simulink model "Main"  (R2023a)
settings: Solver=ode4  StartTime=0.0  StopTime=inf  FixedStep=1e-5  RelTol=1e-3
libraries: canoelib x39, spsControlledVoltageSourceLib x3, spsCurrentMeasurementLib x3, slpidlib x2, vehdynlibsteering x1, spsPermanentMagnetSynchronousMachineLib x1, sps_lib x1, dspnetwork x1, etargetslib x1
settings Model: targetArch=x86  analysisModel=0  XcpMessageLength=-1  hasCAPLCallBlock=0  Creator=hatep  LastModifiedBy=hatep
settings RTWCC: Description=Vector CANoe Real-Time Target DLL (Visual C/C++ Project Makefile)  SystemTargetFile=cn.tlc  TemplateMakefile=cn_msdll.tmf
settings STFCustomTargetCC: ConcurrentExecutionCompliant=off  MatFileLogging=on  UseToolchainInfoCompliant=off  SystemTargetFile=cn.tlc
settings GRTTargetCC: ParMdlRefBuildCompliant=off  CompOptLevelCompliant=off  ConcurrentExecutionCompliant=off  CombineOutputUpdateFcns=off  CPPClassGenCompliant=off  GRTInterface=on  UseToolchainInfoCompliant=off  RTWCAPISignals=on  RTWCAPIParams=on

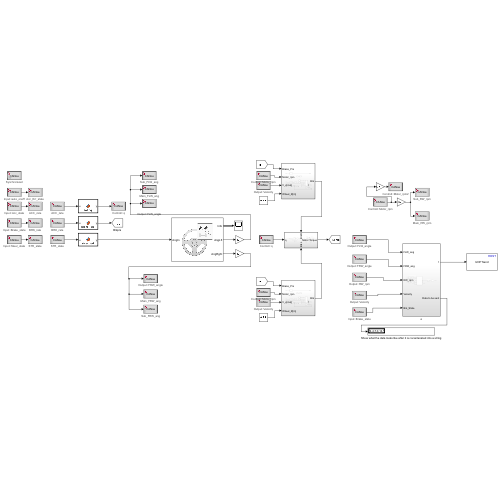
[thumbnail: Simulink's stored preview of the top-level diagram]
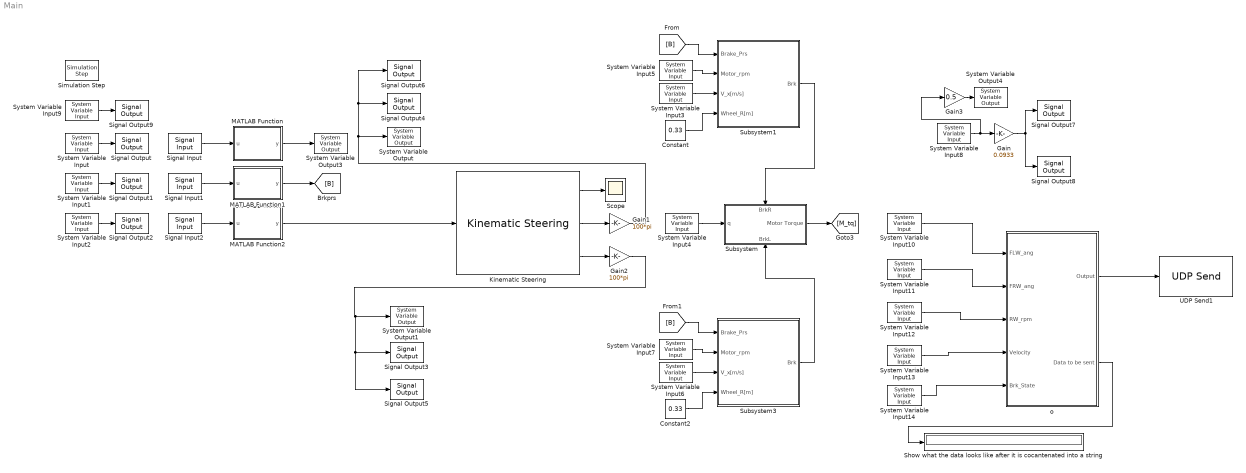
== system Main ==
  Constant : Constant  Value=0.33
  Constant2 : Constant  Value=0.33
  Gain : Gain  Gain=0.0933
  Gain1 : Gain  Gain=100*pi
  Gain2 : Gain  Gain=100*pi
  Gain3 : Gain  Gain=0.5
  Kinematic Steering : vehdynlibsteering/Kinematic Steering  StrgType=Ackerman  StrgRatioType=Constant  Loc=Front  NrmlFctr=1  TrckWdth=3  WhlBase=1.6  Db=0  StrgRng=3*pi  StrgAngBpts="[-6.2832   -5.0265   -3.7699   -2.5133   -1.2566         0    1.2566    2.5133    3.7699    5.0265    6.2832]"  StrgRatioTbl=|  StrgRatio=100  PctAckIn=off  PctAck=100  PctAckTbl=ones(1,11)*100  StrgArmLngth=0.1  RckCsLngth=0.5  TieRodLngth=0.248  D=0.2  PnnRadius=0.00085818  PnnRadiusTbl="[0.0055    0.0055    0.0056    0.0057    0.0058    0.0057    0.0057    0.0057    0.0056    0.0055    0.0055]"  RodLngth=0.1  ParaArmLngth=0.9  aMode=2
      | [13.5000   13.3750   13.2500   13.1250   13.0000   13.0000   13.0000   13.1250   13.2500   13.3750   13.5000
      | ]
  MATLAB Function : MATLAB Function  TreatAsAtomicUnit=on
  MATLAB Function1 : MATLAB Function  TreatAsAtomicUnit=on
  MATLAB Function2 : MATLAB Function  TreatAsAtomicUnit=on
  Scope : Scope
  Show what the data looks like after it is cocantenated into a string : Display
  Signal Input : canoelib/CANoe I//O/Signal Input  dbName=MBD  nodeName=Veh_Sim  msgName=Sim_1  sigName=ACC_rate  editSampleTime=0  rawValue=Default  dataType=Default  dataTypeDB=uint8  hasEncoding=off
      settings: AttributesFormatString=%<sigName>  SourceProductName=Vector CANoe
  Signal Input1 : canoelib/CANoe I//O/Signal Input  dbName=MBD  nodeName=Veh_Sim  msgName=Sim_1  sigName=BRK_rate  editSampleTime=0  rawValue=Default  dataType=Default  dataTypeDB=uint8  hasEncoding=off
      settings: AttributesFormatString=%<sigName>  SourceProductName=Vector CANoe
  Signal Input2 : canoelib/CANoe I//O/Signal Input  dbName=MBD  nodeName=Veh_Sim  msgName=Sim_1  sigName=STR_state  editSampleTime=0  rawValue=Default  dataType=Default  dataTypeDB=int8  hasEncoding=off
      settings: AttributesFormatString=%<sigName>  SourceProductName=Vector CANoe
  Signal Output : canoelib/CANoe I//O/Signal Output  dbName=MBD  nodeName=Veh_Sim  msgName=Sim_1  sigName=ACC_rate  rawValue=Default  dataType=Default  dataTypeDB=uint8  hasEncoding=off
      settings: AttributesFormatString=%<sigName>  SourceProductName=Vector CANoe
  Signal Output1 : canoelib/CANoe I//O/Signal Output  dbName=MBD  nodeName=Veh_Sim  msgName=Sim_1  sigName=BRK_rate  rawValue=Default  dataType=Default  dataTypeDB=uint8  hasEncoding=off
      settings: AttributesFormatString=%<sigName>  SourceProductName=Vector CANoe
  Signal Output2 : canoelib/CANoe I//O/Signal Output  dbName=MBD  nodeName=Veh_Sim  msgName=Sim_1  sigName=STR_state  rawValue=Default  dataType=Default  dataTypeDB=int8  hasEncoding=off
      settings: AttributesFormatString=%<sigName>  SourceProductName=Vector CANoe
  Signal Output3 : canoelib/CANoe I//O/Signal Output  dbName=MBD  nodeName=MainCtr  msgName=Ctr  sigName=Main_FRW_ang  rawValue=Raw value  dataType=Default  dataTypeDB=int8  hasEncoding=off
      settings: AttributesFormatString=%<sigName>  SourceProductName=Vector CANoe
  Signal Output4 : canoelib/CANoe I//O/Signal Output  dbName=MBD  nodeName=MainCtr  msgName=Ctr  sigName=Main_FLW_ang  rawValue=Raw value  dataType=Default  dataTypeDB=int8  hasEncoding=off
      settings: AttributesFormatString=%<sigName>  SourceProductName=Vector CANoe
  Signal Output5 : canoelib/CANoe I//O/Signal Output  dbName=MBD  nodeName=SubCtr  msgName=Sub_Ctr  sigName=Sub_FRW_ang  rawValue=Raw value  dataType=Default  dataTypeDB=uint8  hasEncoding=off
      settings: AttributesFormatString=%<sigName>  SourceProductName=Vector CANoe
  Signal Output6 : canoelib/CANoe I//O/Signal Output  dbName=MBD  nodeName=SubCtr  msgName=Sub_Ctr  sigName=Sub_FLW_ang  rawValue=Raw value  dataType=Default  dataTypeDB=uint8  hasEncoding=on
      settings: AttributesFormatString=%<sigName>  SourceProductName=Vector CANoe
  Signal Output7 : canoelib/CANoe I//O/Signal Output  dbName=MBD  nodeName=SubCtr  msgName=Sub_Ctr  sigName=Sub_RW_rpm  rawValue=Raw value  dataType=Default  dataTypeDB=uint16  hasEncoding=off
      settings: AttributesFormatString=%<sigName>  SourceProductName=Vector CANoe
  Signal Output8 : canoelib/CANoe I//O/Signal Output  dbName=MBD  nodeName=MainCtr  msgName=Ctr  sigName=Main_RW_rpm  rawValue=Raw value  dataType=Default  dataTypeDB=uint16  hasEncoding=off
      settings: AttributesFormatString=%<sigName>  SourceProductName=Vector CANoe
  Signal Output9 : canoelib/CANoe I//O/Signal Output  dbName=MBD  nodeName=Veh_Sim  msgName=Accel_Error_Condition  sigName=Acc_Err_state  rawValue=Default  dataType=Default  dataTypeDB=boolean  hasEncoding=off
      settings: AttributesFormatString=%<sigName>  SourceProductName=Vector CANoe
  Simulation Step : canoelib/CANoe I//O/Simulation Step  mode=Synchronized
      settings: AttributesFormatString=%<mode>  SourceProductName=Vector CANoe
  Subsystem : Subsystem
      settings: PortSchema="{\"entries\":[{\"content\":{\"sides\":[{\"content\":{\"connectorIds\":[\"In1\"]},\"type\":\"ConnectorPlacement.EquallySpacedRectSide\",\"uuid\":\"d856fc92-af2a-46c6-aa2d-f38a71ec206d\"},{\"content\":{\"connectorIds\":[\"Out1\"],\"side\":\"RIGHT\"},\"type\":\"ConnectorPlacement.EquallySpacedRectSide\",\"uuid\":\"749cbdd8-772b-4c60-b55a-bc78d69c198e\"},{\"content\":{\"connectorIds\":[\"In2\"],\"side\":\"TOP\"},\"type\":\"ConnectorPlacement.EquallySpacedRectSide\",\"uuid\":\"8a4e4948-29bd-4e64-b879-f0ed3d2cb3aa\"},{\"content\":{\"connectorIds\":[\"In3\"],\"side\":\"BOTTOM\"},\"type\":\"ConnectorPlacement.EquallySpacedRectSide\",\"uuid\":\"fb5f1ea8-5bd9-47f7-a40f-d5738de871d9\"}]},\"type\":\"ConnectorPlacement.EquallySpacedConnector\",\"uuid\":\"7c29b0f2-06f1-46e9-896a-7c6ebac9527c\"}],\"packageUris\":[\"http://schema.mathworks.com/mf0/Connector/R2020b\"],\"version\":\"1.0\"}"
  Subsystem1 : Subsystem
  Subsystem3 : Subsystem
  System Variable Input : canoelib/CANoe I//O/System Variable Input  nsName=Input  sysVarName=Acc_state  arrayIndex=-1  editSampleTime=0  rawValue=Default  dataType=Default  dataTypeDB=int32  hasEncoding=off  dataTypeCANoe=Get from CANoe
      settings: AttributesFormatString=%<nsName>::%<sysVarName>  SourceProductName=Vector CANoe
  System Variable Input1 : canoelib/CANoe I//O/System Variable Input  nsName=Input  sysVarName=Brake_state  arrayIndex=-1  editSampleTime=0  rawValue=Default  dataType=Default  dataTypeDB=int32  hasEncoding=off  dataTypeCANoe=Get from CANoe
      settings: AttributesFormatString=%<nsName>::%<sysVarName>  SourceProductName=Vector CANoe
  System Variable Input10 : canoelib/CANoe I//O/System Variable Input  nsName=Output  sysVarName=FLW_angle  arrayIndex=-1  editSampleTime=0  rawValue=Default  dataType=Default  dataTypeDB=int32  hasEncoding=off  dataTypeCANoe=Get from CANoe
      settings: AttributesFormatString=%<nsName>::%<sysVarName>  SourceProductName=Vector CANoe
  System Variable Input11 : canoelib/CANoe I//O/System Variable Input  nsName=Output  sysVarName=FRW_angle  arrayIndex=-1  editSampleTime=0  rawValue=Default  dataType=Default  dataTypeDB=int32  hasEncoding=off  dataTypeCANoe=Get from CANoe
      settings: AttributesFormatString=%<nsName>::%<sysVarName>  SourceProductName=Vector CANoe
  System Variable Input12 : canoelib/CANoe I//O/System Variable Input  nsName=Output  sysVarName=RW_rpm  arrayIndex=-1  editSampleTime=0  rawValue=Default  dataType=Default  dataTypeDB=int32  hasEncoding=off  dataTypeCANoe=Get from CANoe
      settings: AttributesFormatString=%<nsName>::%<sysVarName>  SourceProductName=Vector CANoe
  System Variable Input13 : canoelib/CANoe I//O/System Variable Input  nsName=Output  sysVarName=Velocity  arrayIndex=-1  editSampleTime=0  rawValue=Default  dataType=Default  dataTypeDB=int32  hasEncoding=off  dataTypeCANoe=Get from CANoe
      settings: AttributesFormatString=%<nsName>::%<sysVarName>  SourceProductName=Vector CANoe
  System Variable Input14 : canoelib/CANoe I//O/System Variable Input  nsName=Input  sysVarName=Brake_state  arrayIndex=-1  editSampleTime=0  rawValue=Default  dataType=Default  dataTypeDB=int32  hasEncoding=off  dataTypeCANoe=Get from CANoe
      settings: AttributesFormatString=%<nsName>::%<sysVarName>  SourceProductName=Vector CANoe
  System Variable Input2 : canoelib/CANoe I//O/System Variable Input  nsName=Input  sysVarName=Steer_state  arrayIndex=-1  editSampleTime=0  rawValue=Default  dataType=Default  dataTypeDB=int32  hasEncoding=off  dataTypeCANoe=Get from CANoe
      settings: AttributesFormatString=%<nsName>::%<sysVarName>  SourceProductName=Vector CANoe
  System Variable Input3 : canoelib/CANoe I//O/System Variable Input  nsName=Output  sysVarName=Velocity  arrayIndex=-1  editSampleTime=0  rawValue=Default  dataType=Default  dataTypeDB=int32  hasEncoding=off  dataTypeCANoe=Get from CANoe
      settings: AttributesFormatString=%<nsName>::%<sysVarName>  SourceProductName=Vector CANoe
  System Variable Input4 : canoelib/CANoe I//O/System Variable Input  nsName=Controll  sysVarName=q  arrayIndex=-1  editSampleTime=0  rawValue=Default  dataType=Default  dataTypeDB=double  hasEncoding=off  dataTypeCANoe=Get from CANoe
      settings: AttributesFormatString=%<nsName>::%<sysVarName>  SourceProductName=Vector CANoe
  System Variable Input5 : canoelib/CANoe I//O/System Variable Input  nsName=Controll  sysVarName=Motor_rpm  arrayIndex=-1  editSampleTime=0  rawValue=Default  dataType=Default  dataTypeDB=int32  hasEncoding=off  dataTypeCANoe=Get from CANoe
      settings: AttributesFormatString=%<nsName>::%<sysVarName>  SourceProductName=Vector CANoe
  System Variable Input6 : canoelib/CANoe I//O/System Variable Input  nsName=Output  sysVarName=Velocity  arrayIndex=-1  editSampleTime=0  rawValue=Default  dataType=Default  dataTypeDB=int32  hasEncoding=off  dataTypeCANoe=Get from CANoe
      settings: AttributesFormatString=%<nsName>::%<sysVarName>  SourceProductName=Vector CANoe
  System Variable Input7 : canoelib/CANoe I//O/System Variable Input  nsName=Controll  sysVarName=Motor_rpm  arrayIndex=-1  editSampleTime=0  rawValue=Default  dataType=Default  dataTypeDB=int32  hasEncoding=off  dataTypeCANoe=Get from CANoe
      settings: AttributesFormatString=%<nsName>::%<sysVarName>  SourceProductName=Vector CANoe
  System Variable Input8 : canoelib/CANoe I//O/System Variable Input  nsName=Controll  sysVarName=Motor_rpm  arrayIndex=-1  editSampleTime=0  rawValue=Default  dataType=Default  dataTypeDB=int32  hasEncoding=off  dataTypeCANoe=Get from CANoe
      settings: AttributesFormatString=%<nsName>::%<sysVarName>  SourceProductName=Vector CANoe
  System Variable Input9 : canoelib/CANoe I//O/System Variable Input  nsName=Input  sysVarName=auto_onoff  arrayIndex=-1  editSampleTime=0  rawValue=Default  dataType=Default  dataTypeDB=int32  hasEncoding=off  dataTypeCANoe=Get from CANoe
      settings: AttributesFormatString=%<nsName>::%<sysVarName>  SourceProductName=Vector CANoe
  System Variable Output : canoelib/CANoe I//O/System Variable Output  nsName=Output  sysVarName=FLW_angle  arrayIndex=-1  rawValue=Raw value  dataType=Default  dataTypeDB=int32  hasEncoding=off  dataTypeCANoe=Get from CANoe
      settings: AttributesFormatString=%<nsName>::%<sysVarName>  SourceProductName=Vector CANoe
  System Variable Output1 : canoelib/CANoe I//O/System Variable Output  nsName=Output  sysVarName=FRW_angle  arrayIndex=-1  rawValue=Raw value  dataType=Default  dataTypeDB=int32  hasEncoding=off  dataTypeCANoe=Get from CANoe
      settings: AttributesFormatString=%<nsName>::%<sysVarName>  SourceProductName=Vector CANoe
  System Variable Output3 : canoelib/CANoe I//O/System Variable Output  nsName=Controll  sysVarName=q  arrayIndex=-1  rawValue=Default  dataType=Default  dataTypeDB=double  hasEncoding=off  dataTypeCANoe=Get from CANoe
      settings: AttributesFormatString=%<nsName>::%<sysVarName>  SourceProductName=Vector CANoe
  System Variable Output4 : canoelib/CANoe I//O/System Variable Output  nsName=Controll  sysVarName=Motor_rpm2  arrayIndex=-1  rawValue=Raw value  dataType=Default  dataTypeDB=int32  hasEncoding=off  dataTypeCANoe=Get from CANoe
      settings: AttributesFormatString=%<nsName>::%<sysVarName>  SourceProductName=Vector CANoe
  UDP Send1 : dspnetwork/UDP Send  remoteURL='127.0.0.1'  remotePort=25000  localURL='0.0.0.0'  localPortSource=Automatically determine  localPort=-1  sendBufferSize=8192  sampletime=-1  blockPlatform=HOST  separateLengthPort=0
  o : Subsystem
  wires:
  MATLAB Function/1(y) -> System Variable Output3/1
  MATLAB Function1/1(y) -> [B]
  Kinematic Steering/2 -> Gain1/1
  Kinematic Steering/3 -> Gain2/1
  Kinematic Steering/1 -> Scope/1
  MATLAB Function2/1(y) -> Kinematic Steering/1
  System Variable Input/1 -> Signal Output/1
  Signal Input/1 -> MATLAB Function/1(u)
  Signal Input1/1 -> MATLAB Function1/1(u)
  Signal Input2/1 -> MATLAB Function2/1(u)
  System Variable Input1/1 -> Signal Output1/1
  System Variable Input2/1 -> Signal Output2/1
  Gain1/1 -> Signal Output6/1, Signal Output4/1, System Variable Output/1
  Gain2/1 -> Signal Output5/1, Signal Output3/1, System Variable Output1/1
  System Variable Input4/1 -> Subsystem/1(q)
  Subsystem/1(Motor Torque) -> [M_tq]
  Constant/1 -> Subsystem1/4(Wheel_R[m])
  [B] -> Subsystem1/1(Brake_Prs)
  System Variable Input3/1 -> Subsystem1/3(V_x[m/s])
  System Variable Input5/1 -> Subsystem1/2(Motor_rpm)
  Subsystem1/1(Brk) -> Subsystem/2(BrkR)
  System Variable Input7/1 -> Subsystem3/2(Motor_rpm)
  System Variable Input6/1 -> Subsystem3/3(V_x[m/s])
  [B] -> Subsystem3/1(Brake_Prs)
  Constant2/1 -> Subsystem3/4(Wheel_R[m])
  Subsystem3/1(Brk) -> Subsystem/3(BrkL)
  System Variable Input8/1 -> Gain3/1, Gain/1
  Gain/1 -> Signal Output7/1, Signal Output8/1
  Gain3/1 -> System Variable Output4/1
  o/1(Output) -> UDP Send1/1
  o/2(Data to be sent) -> Show what the data looks like after it is cocantenated into a string/1
  System Variable Input10/1 -> o/1(FLW_ang)
  System Variable Input11/1 -> o/2(FRW_ang)
  System Variable Input12/1 -> o/3(RW_rpm)
  System Variable Input13/1 -> o/4(Velocity)
  System Variable Input14/1 -> o/5(Brk_State)
  System Variable Input9/1 -> Signal Output9/1

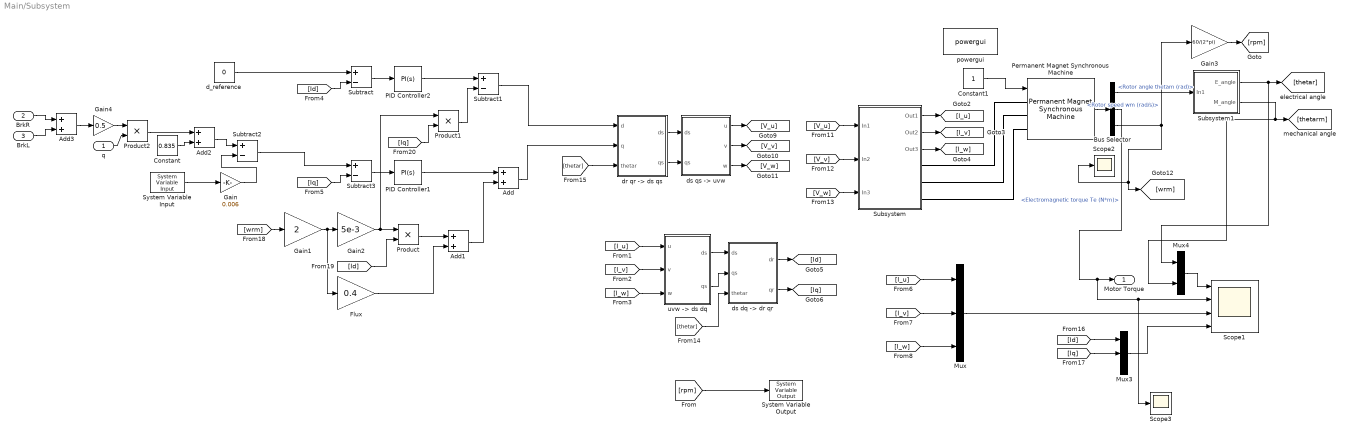
== system Main/Subsystem ==
  q : Inport
  BrkR : Inport  Port=2
  BrkL : Inport  Port=3
  Add{,1..3} (4 alike) : Sum
  Bus Selector : BusSelector  OutputSignals=Rotor angle thetam (rad),Electromagnetic torque Te (N*m),Rotor speed wm (rad/s)
  Constant : Constant  Value=0.835
  Constant1 : Constant
  Flux : Gain  Gain=0.4
  Gain : Gain  Gain=0.006
  Gain1 : Gain  Gain=2
  Gain2 : Gain  Gain=5e-3
  Gain3 : Gain  Gain=60/(2*pi)
  Gain4 : Gain  Gain=0.5
  Mux : Mux  Inputs=3
  Mux3 : Mux  Inputs=3
  Mux4 : Mux  Inputs=2
  PID Controller1 : slpidlib/PID Controller  Controller=PI  Form=Parallel  TimeDomain=Continuous-time  UseExternalTs=off  SampleTime=-1  IntegratorMethod=Forward Euler  FilterMethod=Forward Euler  ControllerParametersSource=internal  P=0.005*500*2*pi  I=0.5*500*2*pi  UseKiTs=off  D=0  N=100  UseFilter=on  TunerSelectOption=Transfer Function Based (PID Tuner App)  InitialConditionSource=internal  InitialConditionForIntegrator=0  InitialConditionForFilter=0  DifferentiatorICPrevScaledInput=0  ExternalReset=none  TrackingMode=off  Kt=1  LimitOutput=off  SatLimitsSource=internal  UpperSaturationLimit=inf  LowerSaturationLimit=-inf  LinearizeAsGain=on  AntiWindupMode=none  Kb=1  LimitIntegrator=off  UpperIntegratorSaturationLimit=inf  LowerIntegratorSaturationLimit=-inf  POutMin=[]  POutMax=[]  IOutMin=[]  IOutMax=[]  DOutMin=[]  DOutMax=[]  NOutMin=[]  NOutMax=[]  SumOutMin=[]  SumOutMax=[]  SaturationOutMin=[]  SaturationOutMax=[]  PParamMin=[]  PParamMax=[]  IParamMin=[]  IParamMax=[]  DParamMin=[]  DParamMax=[]  NParamMin=[]  NParamMax=[]  KbParamMin=[]  KbParamMax=[]  KtParamMin=[]  KtParamMax=[]  KbOutMin=[]  KbOutMax=[]  KtOutMin=[]  KtOutMax=[]  IntegratorOutMin=[]  IntegratorOutMax=[]  FilterOutMin=[]  FilterOutMax=[]  SumI1OutMin=[]  SumI1OutMax=[]  SumI2OutMin=[]  SumI2OutMax=[]  SumI3OutMin=[]  SumI3OutMax=[]  SumI4OutMin=[]  SumI4OutMax=[]  SumDOutMin=[]  SumDOutMax=[]  DifferentiatorOutMin=[]  DifferentiatorOutMax=[]  FilterDiffOutCoefMin=[]  FilterDiffOutCoefMax=[]  ReciprocalOutMin=[]  ReciprocalOutMax=[]  SumDenOutMin=[]  SumDenOutMax=[]  SumNumOutMin=[]  SumNumOutMax=[]  DivideOutMin=[]  DivideOutMax=[]  UdiffTsProdOutMin=[]  UdiffTsProdOutMax=[]  NTsProdOutMin=[]  NTsProdOutMax=[]  UintegralTsProdOutMin=[]  UintegralTsProdOutMax=[]  UngainTsProdOutMin=[]  UngainTsProdOutMax=[]  ClampingZeroOutDataTypeStr=Inherit: Inherit via back propagation  ClampingZeroOutMin=[]  ClampingZeroOutMax=[]  FilterDenConstantOutDataTypeStr=Inherit: Inherit via back propagation  FilterDenConstantOutMin=[]  FilterDenConstantOutMax=[]  PCopyOutDataTypeStr=Inherit: Inherit via back propagation  PCopyOutMin=[]  PCopyOutMax=[]  NCopyOutDataTypeStr=Inherit: Inherit via back propagation  NCopyOutMin=[]  NCopyOutMax=[]  IntegratorContinuousStateAttributes=''  IntegratorStateMustResolveToSignalObject=off  IntegratorRTWStateStorageClass=Auto  FilterContinuousStateAttributes=''  FilterStateMustResolveToSignalObject=off  FilterRTWStateStorageClass=Auto  ParallelPVariant=InternalParameters  IdealPVariant=Disabled  IVariant=InternalParameters  DVariant=Disabled  IntegratorVariant=Continuous  SatVariant=Disabled  AWVariant=Passthrough  PCopyVariant=Disabled  TRVariant=Disabled  FdbkBlocksVariant=Forward  IdealPFdbkVariant=Disabled  SatFdbkVariant=Disabled  DerivativeFilterVariant=Disabled  NVariant=Disabled  NCopyVariant=Disabled_SignalSpec  FilterICVariant=Disabled  IntegratorICVariant=InternalICs  ExternalResetVariant=Disabled  TRSumVariant=Passthrough  SumFdbkVariant=Disabled  SumVariant=Sum_PI  TsampFilterVariant=InternalTs  TsampNgainVariant=Passthrough  TsampIntegralVariant=Disabled_SignalSpec  ExternalSaturationOutDataTypeStr=Inherit: Same as second input
  PID Controller2 : slpidlib/PID Controller  Controller=PI  Form=Parallel  TimeDomain=Continuous-time  UseExternalTs=off  SampleTime=-1  IntegratorMethod=Forward Euler  FilterMethod=Forward Euler  ControllerParametersSource=internal  P=0.005*500*2*pi  I=0.5*500*2*pi  UseKiTs=off  D=0  N=100  UseFilter=on  TunerSelectOption=Transfer Function Based (PID Tuner App)  InitialConditionSource=internal  InitialConditionForIntegrator=0  InitialConditionForFilter=0  DifferentiatorICPrevScaledInput=0  ExternalReset=none  TrackingMode=off  Kt=1  LimitOutput=off  SatLimitsSource=internal  UpperSaturationLimit=inf  LowerSaturationLimit=-inf  LinearizeAsGain=on  AntiWindupMode=none  Kb=1  LimitIntegrator=off  UpperIntegratorSaturationLimit=inf  LowerIntegratorSaturationLimit=-inf  POutMin=[]  POutMax=[]  IOutMin=[]  IOutMax=[]  DOutMin=[]  DOutMax=[]  NOutMin=[]  NOutMax=[]  SumOutMin=[]  SumOutMax=[]  SaturationOutMin=[]  SaturationOutMax=[]  PParamMin=[]  PParamMax=[]  IParamMin=[]  IParamMax=[]  DParamMin=[]  DParamMax=[]  NParamMin=[]  NParamMax=[]  KbParamMin=[]  KbParamMax=[]  KtParamMin=[]  KtParamMax=[]  KbOutMin=[]  KbOutMax=[]  KtOutMin=[]  KtOutMax=[]  IntegratorOutMin=[]  IntegratorOutMax=[]  FilterOutMin=[]  FilterOutMax=[]  SumI1OutMin=[]  SumI1OutMax=[]  SumI2OutMin=[]  SumI2OutMax=[]  SumI3OutMin=[]  SumI3OutMax=[]  SumI4OutMin=[]  SumI4OutMax=[]  SumDOutMin=[]  SumDOutMax=[]  DifferentiatorOutMin=[]  DifferentiatorOutMax=[]  FilterDiffOutCoefMin=[]  FilterDiffOutCoefMax=[]  ReciprocalOutMin=[]  ReciprocalOutMax=[]  SumDenOutMin=[]  SumDenOutMax=[]  SumNumOutMin=[]  SumNumOutMax=[]  DivideOutMin=[]  DivideOutMax=[]  UdiffTsProdOutMin=[]  UdiffTsProdOutMax=[]  NTsProdOutMin=[]  NTsProdOutMax=[]  UintegralTsProdOutMin=[]  UintegralTsProdOutMax=[]  UngainTsProdOutMin=[]  UngainTsProdOutMax=[]  ClampingZeroOutDataTypeStr=Inherit: Inherit via back propagation  ClampingZeroOutMin=[]  ClampingZeroOutMax=[]  FilterDenConstantOutDataTypeStr=Inherit: Inherit via back propagation  FilterDenConstantOutMin=[]  FilterDenConstantOutMax=[]  PCopyOutDataTypeStr=Inherit: Inherit via back propagation  PCopyOutMin=[]  PCopyOutMax=[]  NCopyOutDataTypeStr=Inherit: Inherit via back propagation  NCopyOutMin=[]  NCopyOutMax=[]  IntegratorContinuousStateAttributes=''  IntegratorStateMustResolveToSignalObject=off  IntegratorRTWStateStorageClass=Auto  FilterContinuousStateAttributes=''  FilterStateMustResolveToSignalObject=off  FilterRTWStateStorageClass=Auto  ParallelPVariant=InternalParameters  IdealPVariant=Disabled  IVariant=InternalParameters  DVariant=Disabled  IntegratorVariant=Continuous  SatVariant=Disabled  AWVariant=Passthrough  PCopyVariant=Disabled  TRVariant=Disabled  FdbkBlocksVariant=Forward  IdealPFdbkVariant=Disabled  SatFdbkVariant=Disabled  DerivativeFilterVariant=Disabled  NVariant=Disabled  NCopyVariant=Disabled_SignalSpec  FilterICVariant=Disabled  IntegratorICVariant=InternalICs  ExternalResetVariant=Disabled  TRSumVariant=Passthrough  SumFdbkVariant=Disabled  SumVariant=Sum_PI  TsampFilterVariant=InternalTs  TsampNgainVariant=Passthrough  TsampIntegralVariant=Disabled_SignalSpec  ExternalSaturationOutDataTypeStr=Inherit: Same as second input
  Permanent Magnet Synchronous Machine : spsPermanentMagnetSynchronousMachineLib/Permanent Magnet Synchronous Machine  NbPhases=3  FluxDistribution=Sinusoidal  RotorType=Round  MechanicalLoad=Torque Tm  PresetModel=No  ShowDetailedParameters=on  MeasurementBus=off  Resistance=0.5  Inductance=8.5e-3  dqInductances=[8.5e-3,8.5e-3]  La=0.005  MachineConstant=Flux linkage established by magnets (V.s)  Flux=0.4  VoltageCst=145.1039  TorqueCst=1.2  Flat=120  Mechanical=[0.003 0.004 2 0]  PolePairs=4  InitialConditions=[0,0, 0,0]  InitialConditions5ph=[0 0 0 0 0 0]  RefAngle=Aligned with phase A axis (original Park)  IterativeDiscreteModel=Trapezoidal non iterative  TsBlock=-1  TsPowergui=0
  Product : Product
  Product1 : Product
  Product2 : Product
  Scope1 : Scope  NumInputPorts=4
  Scope2 : Scope
  Scope3 : Scope
  Subsystem : Subsystem
  Subsystem1 : Subsystem
  Subtract{,1..3} (4 alike) : Sum  Inputs=+-
  System Variable Input : canoelib/CANoe I//O/System Variable Input  nsName=Controll  sysVarName=Motor_rpm  arrayIndex=-1  editSampleTime=0  rawValue=Default  dataType=Default  dataTypeDB=int32  hasEncoding=off  dataTypeCANoe=Get from CANoe
      settings: AttributesFormatString=%<nsName>::%<sysVarName>  SourceProductName=Vector CANoe
  System Variable Output : canoelib/CANoe I//O/System Variable Output  nsName=Controll  sysVarName=Motor_rpm  arrayIndex=-1  rawValue=Default  dataType=Default  dataTypeDB=int32  hasEncoding=off  dataTypeCANoe=Get from CANoe
      settings: AttributesFormatString=%<nsName>::%<sysVarName>  SourceProductName=Vector CANoe
  d_reference : Constant  Value=0
  "dr qr -> ds qs" : Subsystem
  "ds dq -> dr qr" : Subsystem
  "ds qs -> uvw" : Subsystem
  powergui : sps_lib/powergui  Priority=1  SimulationMode=Continuous  SampleTime=50e-6  frequency=60  Iterations=50  frequencyindice=0  Pbase=100e6  ErrMax=1e-4  UnitsV=kV  UnitsW=MW  buscounter=0  FunctionMessages=off  echomessages=off  EnableUseOfTLC=off  CurrentSourceSwitches=off  DisableSnubberDevices=off  DisableRonSwitches=off  DisableVfSwitches=off  DisplayEquations=off  AutomaticDiscreteSolvers=off  SolverType=Tustin/Backward Euler (TBE)  Interpol=off  ExternalGateDelay=off  methode=off  Ts=100  x0status=blocks  SPID=on  SwTol=0  HookPort=off  NonlinearTolerance=1e-4  nMaxIteration=100  ContinueOnMaxIteration=off  RestoreLinks=warning  ResistiveCurrentMeasurement=off  Frange=[0:2:500]  Ylog=off  Xlog=on  ShowGrid=off  save=off  variable=ZData  structure=0  ZoomFFT=off  StartTime=0.0  cycles=1  DisplayStyle=1  fundamental=60  FreqAxis=off  MaxFrequency=1000  frequencyindicesteady=1  RmsSteady=1  display=off
  "uvw -> ds dq" : Subsystem
  Motor Torque : Outport
  wires:
  [rpm] -> System Variable Output/1
  Bus Selector/2 -> Scope3/1, Scope1/2, Motor Torque/1  "<Electromagnetic torque Te (N*m)>"
  Constant1/1 -> Permanent Magnet Synchronous Machine/1
  [Iq] -> Subtract3/2
  d_reference/1 -> Subtract/1
  "uvw -> ds dq"/1(ds) -> "ds dq -> dr qr"/1(ds)
  Subtract3/1 -> PID Controller1/1
  [thetar] -> "ds dq -> dr qr"/3(thetar)
  Product1/1 -> Subtract1/2
  [wrm] -> Gain1/1
  "uvw -> ds dq"/2(qs) -> "ds dq -> dr qr"/2(qs)
  Gain2/1 -> Product1/1, Product/1
  [I_u] -> Mux/1
  [V_w] -> Subsystem/3(In3)
  Subsystem/2(Out2) -> [I_v]
  [Id] -> Product/2
  Subsystem1/1(E_angle) -> Mux4/1, [thetar]
  PID Controller1/1 -> Add/1
  Mux4/1 -> Scope1/1
  "ds qs -> uvw"/1(u) -> [V_u]
  "ds dq -> dr qr"/1(dr) -> [Id]
  Mux/1 -> Scope1/3
  Product/1 -> Add1/1
  Mux3/1 -> Scope1/4
  Add/1 -> "dr qr -> ds qs"/2(q)
  Subtract1/1 -> "dr qr -> ds qs"/1(d)
  [V_u] -> Subsystem/1(In1)
  Flux/1 -> Add1/2
  Add1/1 -> Add/2
  [thetar] -> "dr qr -> ds qs"/3(thetar)
  PID Controller2/1 -> Subtract1/1
  Bus Selector/1 -> Subsystem1/1(In1)  "<Rotor angle thetam (rad)>"
  "dr qr -> ds qs"/1(ds) -> "ds qs -> uvw"/1(ds)
  "ds dq -> dr qr"/2(qr) -> [Iq]
  Subsystem/1(Out1) -> [I_u]
  [I_w] -> Mux/3
  "ds qs -> uvw"/2(v) -> [V_v]
  Bus Selector/3 -> Scope2/1, [wrm], Gain3/1  "<Rotor speed wm (rad/s)>"
  Subsystem/3(Out3) -> [I_w]
  Permanent Magnet Synchronous Machine/1 -> Bus Selector/1
  [Iq] -> Product1/2
  [I_v] -> "uvw -> ds dq"/2(v)
  Subtract/1 -> PID Controller2/1
  [Iq] -> Mux3/2
  Subsystem1/2(M_angle) -> Mux4/2, [thetarm]
  [Id] -> Subtract/2
  [I_u] -> "uvw -> ds dq"/1(u)
  "dr qr -> ds qs"/2(qs) -> "ds qs -> uvw"/2(qs)
  [V_v] -> Subsystem/2(In2)
  [I_w] -> "uvw -> ds dq"/3(w)
  [Id] -> Mux3/1
  "ds qs -> uvw"/3(w) -> [V_w]
  [I_v] -> Mux/2
  Gain3/1 -> [rpm]
  Gain1/1 -> Flux/1, Gain2/1
  q/1 -> Product2/2
  Subtract2/1 -> Subtract3/1
  System Variable Input/1 -> Gain/1
  Gain/1 -> Subtract2/2
  Product2/1 -> Add2/1
  Add2/1 -> Subtract2/1
  Constant/1 -> Add2/2
  BrkL/1 -> Add3/2
  BrkR/1 -> Add3/1
  Add3/1 -> Gain4/1
  Gain4/1 -> Product2/1
  connections:
  Subsystem/RConn1 -- Permanent Magnet Synchronous Machine/LConn1
  Subsystem/RConn3 -- Permanent Magnet Synchronous Machine/LConn3
  Subsystem/RConn2 -- Permanent Magnet Synchronous Machine/LConn2

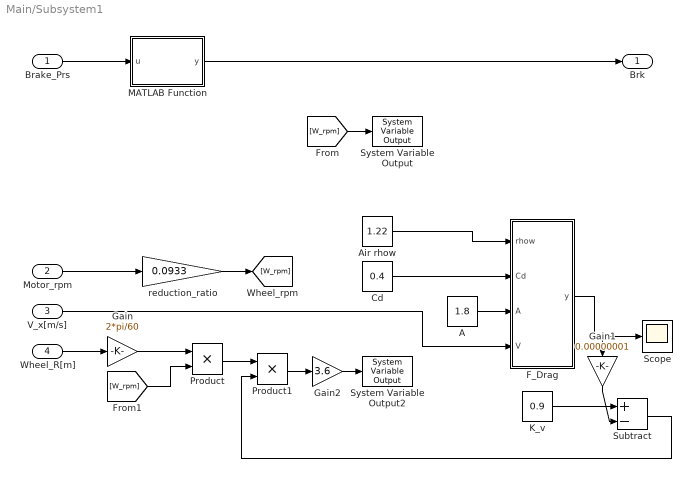
== system Main/Subsystem1 ==
  Brake_Prs : Inport
  Motor_rpm : Inport  Port=2
  V_x[m/s] : Inport  Port=3
  Wheel_R[m] : Inport  Port=4
  A : Constant  Value=1.8
  Air rhow : Constant  Value=1.22
  Cd : Constant  Value=0.4
  F_Drag : MATLAB Function  TreatAsAtomicUnit=on
  Gain : Gain  Gain=2*pi/60
  Gain1 : Gain  Gain=0.00000001
  Gain2 : Gain  Gain=3.6
  K_v : Constant  Value=0.9
  MATLAB Function : MATLAB Function  TreatAsAtomicUnit=on
  Product : Product
  Product1 : Product
  Scope : Scope
  Subtract : Sum  Inputs=+-
  System Variable Output : canoelib/CANoe I//O/System Variable Output  nsName=Output  sysVarName=RW_rpm  arrayIndex=-1  rawValue=Default  dataType=Default  dataTypeDB=int32  hasEncoding=off  dataTypeCANoe=Get from CANoe
      settings: AttributesFormatString=%<nsName>::%<sysVarName>  SourceProductName=Vector CANoe
  System Variable Output2 : canoelib/CANoe I//O/System Variable Output  nsName=Output  sysVarName=Velocity  arrayIndex=-1  rawValue=Default  dataType=Default  dataTypeDB=int32  hasEncoding=off  dataTypeCANoe=Get from CANoe
      settings: AttributesFormatString=%<nsName>::%<sysVarName>  SourceProductName=Vector CANoe
  reduction_ratio : Gain  Gain=0.0933
  Brk : Outport
  wires:
  Motor_rpm/1 -> reduction_ratio/1
  reduction_ratio/1 -> [W_rpm]
  V_x[m/s]/1 -> F_Drag/4(V)
  Air rhow/1 -> F_Drag/1(rhow)
  Cd/1 -> F_Drag/2(Cd)
  A/1 -> F_Drag/3(A)
  [W_rpm] -> System Variable Output/1
  Wheel_R[m]/1 -> Gain/1
  [W_rpm] -> Product/2
  Product/1 -> Product1/1
  K_v/1 -> Subtract/1
  Brake_Prs/1 -> MATLAB Function/1(u)
  Gain/1 -> Product/1
  F_Drag/1(y) -> Scope/1, Gain1/1
  Subtract/1 -> Product1/2
  Product1/1 -> Gain2/1
  Gain1/1 -> Subtract/2
  Gain2/1 -> System Variable Output2/1
  MATLAB Function/1(y) -> Brk/1

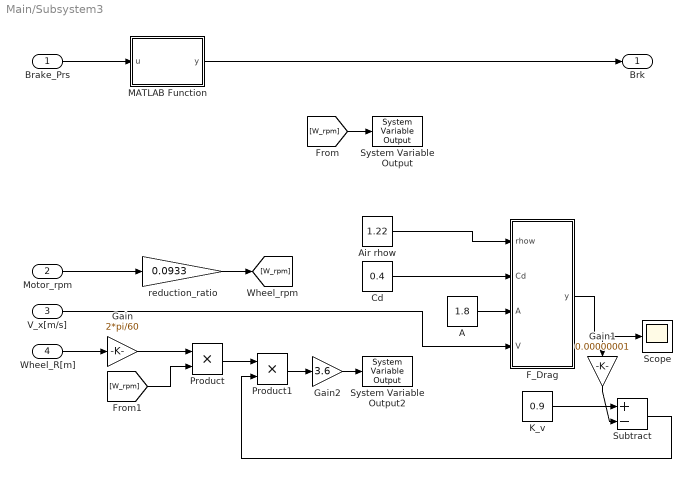
== system Main/Subsystem3 ==
  Brake_Prs : Inport
  Motor_rpm : Inport  Port=2
  V_x[m/s] : Inport  Port=3
  Wheel_R[m] : Inport  Port=4
  A : Constant  Value=1.8
  Air rhow : Constant  Value=1.22
  Cd : Constant  Value=0.4
  F_Drag : MATLAB Function  TreatAsAtomicUnit=on
  Gain : Gain  Gain=2*pi/60
  Gain1 : Gain  Gain=0.00000001
  Gain2 : Gain  Gain=3.6
  K_v : Constant  Value=0.9
  MATLAB Function : MATLAB Function  TreatAsAtomicUnit=on
  Product : Product
  Product1 : Product
  Scope : Scope
  Subtract : Sum  Inputs=+-
  System Variable Output : canoelib/CANoe I//O/System Variable Output  nsName=Output  sysVarName=RW_rpm  arrayIndex=-1  rawValue=Default  dataType=Default  dataTypeDB=int32  hasEncoding=off  dataTypeCANoe=Get from CANoe
      settings: AttributesFormatString=%<nsName>::%<sysVarName>  SourceProductName=Vector CANoe
  System Variable Output2 : canoelib/CANoe I//O/System Variable Output  nsName=Output  sysVarName=Velocity  arrayIndex=-1  rawValue=Default  dataType=Default  dataTypeDB=int32  hasEncoding=off  dataTypeCANoe=Get from CANoe
      settings: AttributesFormatString=%<nsName>::%<sysVarName>  SourceProductName=Vector CANoe
  reduction_ratio : Gain  Gain=0.0933
  Brk : Outport
  wires:
  Motor_rpm/1 -> reduction_ratio/1
  reduction_ratio/1 -> [W_rpm]
  V_x[m/s]/1 -> F_Drag/4(V)
  Air rhow/1 -> F_Drag/1(rhow)
  Cd/1 -> F_Drag/2(Cd)
  A/1 -> F_Drag/3(A)
  [W_rpm] -> System Variable Output/1
  Wheel_R[m]/1 -> Gain/1
  [W_rpm] -> Product/2
  Product/1 -> Product1/1
  K_v/1 -> Subtract/1
  Brake_Prs/1 -> MATLAB Function/1(u)
  Gain/1 -> Product/1
  F_Drag/1(y) -> Scope/1, Gain1/1
  Subtract/1 -> Product1/2
  Product1/1 -> Gain2/1
  Gain1/1 -> Subtract/2
  Gain2/1 -> System Variable Output2/1
  MATLAB Function/1(y) -> Brk/1

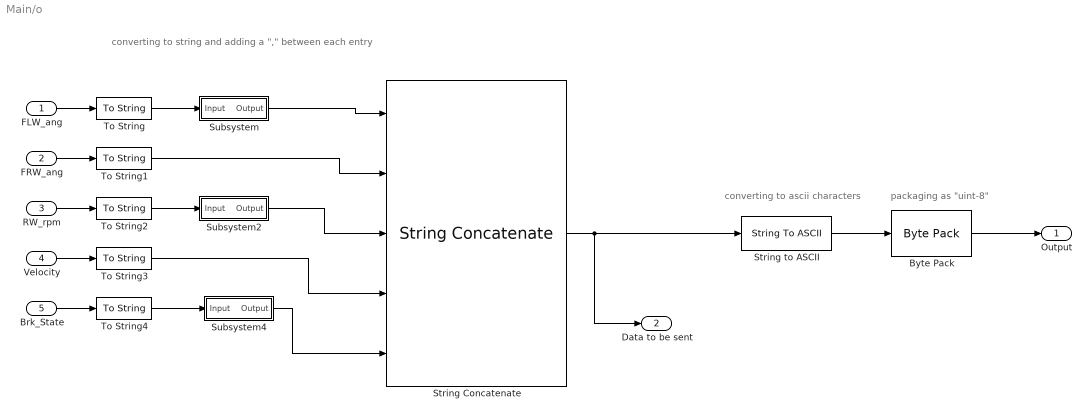
== system Main/o ==
  note: packaging as "uint-8"
  note: converting to ascii characters
  note: converting to string and adding a "," between each entry
  FLW_ang : Inport
  FRW_ang : Inport  Port=2
  RW_rpm : Inport  Port=3
  Velocity : Inport  Port=4
  Brk_State : Inport  Port=5
  Byte Pack : etargetslib/Byte Pack  datatypes={'uint8'}  byteAlign=1
  String Concatenate : StringConcatenate  Inputs=5
  String to ASCII : StringToASCII  OutputVectorSize=64
  Subsystem : Subsystem
  Subsystem2 : Subsystem
  Subsystem4 : Subsystem
  To String{,1..4} (5 alike) : ToString
  Output : Outport
  Data to be sent : Outport  Port=2
  wires:
  String Concatenate/1 -> Data to be sent/1, String to ASCII/1
  To String3/1 -> String Concatenate/4
  To String2/1 -> Subsystem2/1(Input)
  Subsystem4/1(Output) -> String Concatenate/5
  String to ASCII/1 -> Byte Pack/1
  To String/1 -> Subsystem/1(Input)
  Subsystem2/1(Output) -> String Concatenate/3
  To String1/1 -> String Concatenate/2
  To String4/1 -> Subsystem4/1(Input)
  Subsystem/1(Output) -> String Concatenate/1
  Byte Pack/1 -> Output/1
  FRW_ang/1 -> To String1/1
  FLW_ang/1 -> To String/1
  Velocity/1 -> To String3/1
  Brk_State/1 -> To String4/1
  RW_rpm/1 -> To String2/1

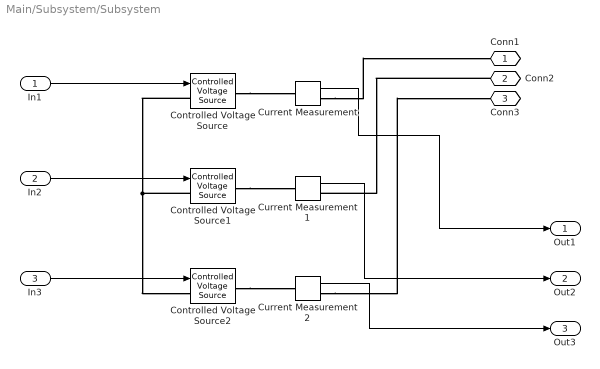
== system Main/Subsystem/Subsystem ==
  In1 : Inport
  In2 : Inport  Port=2
  In3 : Inport  Port=3
  Controlled Voltage Source : spsControlledVoltageSourceLib/Controlled Voltage Source  Initialize=on  Source_Type=AC  Amplitude=0  Phase=0  Frequency=0  Measurements=None
  Controlled Voltage Source1 : spsControlledVoltageSourceLib/Controlled Voltage Source  Initialize=on  Source_Type=AC  Amplitude=0  Phase=0  Frequency=0  Measurements=None
  Controlled Voltage Source2 : spsControlledVoltageSourceLib/Controlled Voltage Source  Initialize=on  Source_Type=AC  Amplitude=0  Phase=0  Frequency=0  Measurements=None
  Current Measurement : spsCurrentMeasurementLib/Current Measurement  PhasorSimulation=off  OutputType=Complex  PSBequivalent=0
  Current Measurement1 : spsCurrentMeasurementLib/Current Measurement  PhasorSimulation=off  OutputType=Complex  PSBequivalent=0
  Current Measurement2 : spsCurrentMeasurementLib/Current Measurement  PhasorSimulation=off  OutputType=Complex  PSBequivalent=0
  Conn1 : PMIOPort  Side=Right
  Conn2 : PMIOPort  Port=2  Side=Right
  Conn3 : PMIOPort  Port=3  Side=Right
  Out1 : Outport
  Out2 : Outport  Port=2
  Out3 : Outport  Port=3
  wires:
  Current Measurement1/1 -> Out2/1
  In3/1 -> Controlled Voltage Source2/1
  In2/1 -> Controlled Voltage Source1/1
  In1/1 -> Controlled Voltage Source/1
  Current Measurement2/1 -> Out3/1
  Current Measurement/1 -> Out1/1
  connections:
  Current Measurement/RConn1 -- Conn1/RConn1
  Controlled Voltage Source/LConn1 -- Controlled Voltage Source1/LConn1 -- Controlled Voltage Source2/LConn1
  Controlled Voltage Source/RConn1 -- Current Measurement/LConn1
  Conn2/RConn1 -- Current Measurement1/RConn1
  Current Measurement2/RConn1 -- Conn3/RConn1
  Controlled Voltage Source1/RConn1 -- Current Measurement1/LConn1
  Controlled Voltage Source2/RConn1 -- Current Measurement2/LConn1

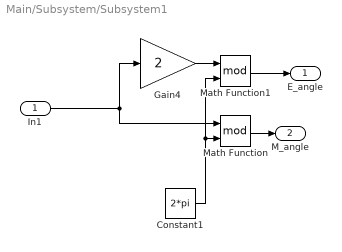
== system Main/Subsystem/Subsystem1 ==
  In1 : Inport
  Constant1 : Constant  Value=2*pi
  Gain4 : Gain  Gain=2
  Math Function : Math  Operator=mod  SignedPower=on
  Math Function1 : Math  Operator=mod  SignedPower=on
  E_angle : Outport
  M_angle : Outport  Port=2
  wires:
  In1/1 -> Gain4/1, Math Function/1
  Constant1/1 -> Math Function1/2, Math Function/2
  Math Function/1 -> M_angle/1
  Gain4/1 -> Math Function1/1
  Math Function1/1 -> E_angle/1

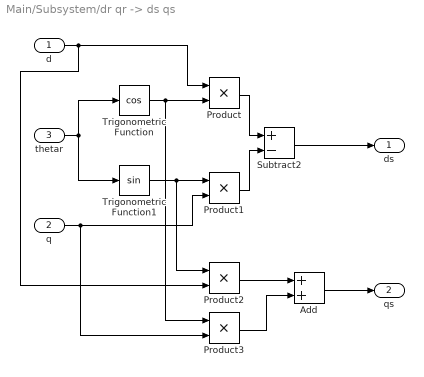
== system Main/Subsystem/dr qr -> ds qs ==
  d : Inport
  q : Inport  Port=2
  thetar : Inport  Port=3
  Add : Sum
  Product{,1..3} (4 alike) : Product
  Subtract2 : Sum  Inputs=+-
  Trigonometric Function : Trigonometry  Operator=cos
  Trigonometric Function1 : Trigonometry
  ds : Outport
  qs : Outport  Port=2
  wires:
  Product3/1 -> Add/2
  Product2/1 -> Add/1
  d/1 -> Product2/2, Product/1
  Add/1 -> qs/1
  Subtract2/1 -> ds/1
  Product1/1 -> Subtract2/2
  Product/1 -> Subtract2/1
  q/1 -> Product1/2, Product3/2
  Trigonometric Function1/1 -> Product1/1, Product2/1
  Trigonometric Function/1 -> Product/2, Product3/1
  thetar/1 -> Trigonometric Function1/1, Trigonometric Function/1

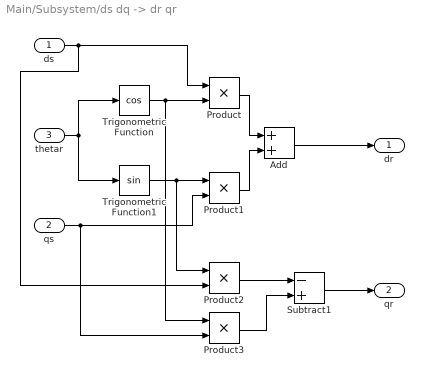
== system Main/Subsystem/ds dq -> dr qr ==
  ds : Inport
  qs : Inport  Port=2
  thetar : Inport  Port=3
  Add : Sum
  Product{,1..3} (4 alike) : Product
  Subtract1 : Sum  Inputs=-+
  Trigonometric Function : Trigonometry  Operator=cos
  Trigonometric Function1 : Trigonometry
  dr : Outport
  qr : Outport  Port=2
  wires:
  thetar/1 -> Trigonometric Function/1, Trigonometric Function1/1
  Trigonometric Function/1 -> Product3/1, Product/2
  Trigonometric Function1/1 -> Product2/1, Product1/1
  qs/1 -> Product3/2, Product1/2
  Product/1 -> Add/1
  Product1/1 -> Add/2
  Add/1 -> dr/1
  Subtract1/1 -> qr/1
  ds/1 -> Product/1, Product2/2
  Product2/1 -> Subtract1/1
  Product3/1 -> Subtract1/2

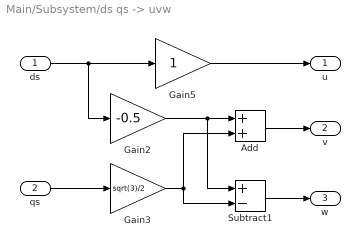
== system Main/Subsystem/ds qs -> uvw ==
  ds : Inport
  qs : Inport  Port=2
  Add : Sum
  Gain2 : Gain  Gain=-0.5
  Gain3 : Gain  Gain=sqrt(3)/2
  Gain5 : Gain
  Subtract1 : Sum  Inputs=+-
  u : Outport
  v : Outport  Port=2
  w : Outport  Port=3
  wires:
  ds/1 -> Gain2/1, Gain5/1
  Gain3/1 -> Subtract1/2, Add/2
  Gain2/1 -> Subtract1/1, Add/1
  Add/1 -> v/1
  Subtract1/1 -> w/1
  qs/1 -> Gain3/1
  Gain5/1 -> u/1

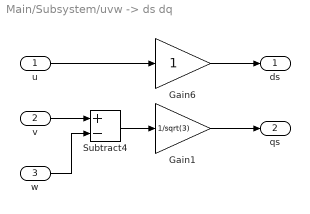
== system Main/Subsystem/uvw -> ds dq ==
  u : Inport
  v : Inport  Port=2
  w : Inport  Port=3
  Gain1 : Gain  Gain=1/sqrt(3)
  Gain6 : Gain
  Subtract4 : Sum  Inputs=+-
  ds : Outport
  qs : Outport  Port=2
  wires:
  v/1 -> Subtract4/1
  u/1 -> Gain6/1
  w/1 -> Subtract4/2
  Gain1/1 -> qs/1
  Subtract4/1 -> Gain1/1
  Gain6/1 -> ds/1

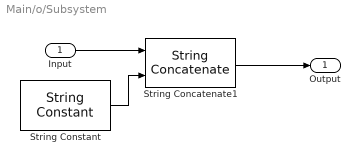
== system Main/o/Subsystem ==
  Input : Inport
  String Concatenate1 : StringConcatenate
  String Constant : StringConstant  String="\",\""
  Output : Outport
  wires:
  Input/1 -> String Concatenate1/1
  String Constant/1 -> String Concatenate1/2
  String Concatenate1/1 -> Output/1

== system Main/o/Subsystem2 ==
  Input : Inport
  String Concatenate1 : StringConcatenate  Inputs=3
  String Constant : StringConstant  String="\",\""
  Output : Outport
  wires:
  String Concatenate1/1 -> Output/1
  Input/1 -> String Concatenate1/2
  String Constant/1 -> String Concatenate1/3, String Concatenate1/1

== system Main/o/Subsystem4 ==
  Input : Inport
  String Concatenate1 : StringConcatenate  Inputs=3
  String Constant : StringConstant  String="\",\""
  Output : Outport
  wires:
  String Concatenate1/1 -> Output/1
  Input/1 -> String Concatenate1/2
  String Constant/1 -> String Concatenate1/3, String Concatenate1/1

== matlab function Main/MATLAB Function1 ==
  data: u input; y output
function y = brake_prs(u)

y = -0.5*(u-15)^2+112.5;

== matlab function Main/MATLAB Function ==
  data: u input; y output
function y= Axltoq(u)

y = -0.25*u^2 + 11.25*u;

== matlab function Main/MATLAB Function2 ==
  data: u input; y output
function y = steer_rad(u)

y = u/254*6*pi;

== matlab function Main/Subsystem1/F_Drag ==
  data: rhow input; y output; Cd input; A input; V input
function y = F_Drag(rhow, Cd,A, V)

y = 0.5*rhow*Cd*A*V^2;

== matlab function Main/Subsystem1/MATLAB Function ==
  data: u input; y output
function y = fcn(u)

y = (112.5-u) / 112.5;

== matlab function Main/Subsystem3/F_Drag ==
  data: rhow input; y output; Cd input; A input; V input
function y = F_Drag(rhow, Cd,A, V)

y = 0.5*rhow*Cd*A*V^2;

== matlab function Main/Subsystem3/MATLAB Function ==
  data: u input; y output
function y = fcn(u)

y = (112.5-u) / 112.5;
